simulink model "InjCtl_qCo1"  (R2016b)
settings: configuration reference "CodeGenConfigSet" (kept outside this file)
values from neighbouring files (symbols this model uses):
  FMA_qCor_C = Calibration.Parameter    [init_InjCtl_qCo.m]    (also in init_InjCtl_qCo_SIL.m = Simulink.Parameter)
  FMO_qCor_C = Calibration.Parameter    [init_InjCtl_qCo.m]    (also in init_InjCtl_qCo_SIL.m = Simulink.Parameter)
  InjCtl_swtDiffQntIn_C = Calibration.Parameter    [init_InjCtl_qCo.m]    (also in init_InjCtl_qCo_SIL.m = Simulink.Parameter)
undefined symbols (not defined in the file or in its folder): EngState_conv, Switch_conv
libraries: simulink x1
settings Model: Creator=lenovo  LastModifiedBy=zhoutinglin
settings ConfigSetRef: SourceLocation=Base Workspace

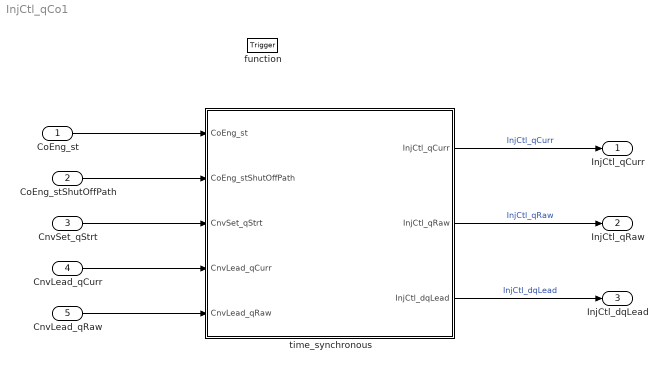
== system InjCtl_qCo1 ==
  CoEng_st : Inport  Description=Engine coordinator state  OutDataTypeStr=Enum: EngState_conv
  CoEng_stShutOffPath : Inport  Description=Active shut-off paths resulting from active reversible,irreversible and afterrun shut-off paths  Port=2  OutMin=0  OutMax=65535  OutDataTypeStr=State_uint16
  CnvSet_qStrt : Inport  Tag=mg/hub  Description=Injection start quantity  Port=3  OutMin=-319  OutMax=319  OutDataTypeStr=FuelMass_mg_hub
  CnvLead_qCurr : Inport  Tag=mg/hub  Description=Injection quantity current path  Port=4  OutMin=-319  OutMax=319  OutDataTypeStr=FuelMass_mg_hub
  CnvLead_qRaw : Inport  Tag=mg/hub  Description=Injection quantity raw path  Port=5  OutMin=-319  OutMax=319  OutDataTypeStr=FuelMass_mg_hub
  function : TriggerPort  TriggerType=function-call  VariantControl=Variant
  time_synchronous : Subsystem
  InjCtl_qCurr : Outport  Tag=mg/hub  Description=Torque generating engine fuel injection quantity  OutMin=-319  OutMax=319  OutDataTypeStr=FuelMass_mg_hub
  InjCtl_qRaw : Outport  Tag=mg/hub  Description=Raw value of injection mass  Port=2  OutMin=-319  OutMax=319  OutDataTypeStr=FuelMass_mg_hub
  InjCtl_dqLead : Outport  Tag=mg/hub  Description=Gradient of quantity  Port=3  OutMin=-319  OutMax=319  OutDataTypeStr=FuelMass_mg_hub
  wires:
  time_synchronous/1(InjCtl_qCurr) -> InjCtl_qCurr/1  "InjCtl_qCurr"
  time_synchronous/2(InjCtl_qRaw) -> InjCtl_qRaw/1  "InjCtl_qRaw"
  time_synchronous/3(InjCtl_dqLead) -> InjCtl_dqLead/1  "InjCtl_dqLead"
  CoEng_st/1 -> time_synchronous/1(CoEng_st)
  CoEng_stShutOffPath/1 -> time_synchronous/2(CoEng_stShutOffPath)
  CnvSet_qStrt/1 -> time_synchronous/3(CnvSet_qStrt)
  CnvLead_qCurr/1 -> time_synchronous/4(CnvLead_qCurr)
  CnvLead_qRaw/1 -> time_synchronous/5(CnvLead_qRaw)

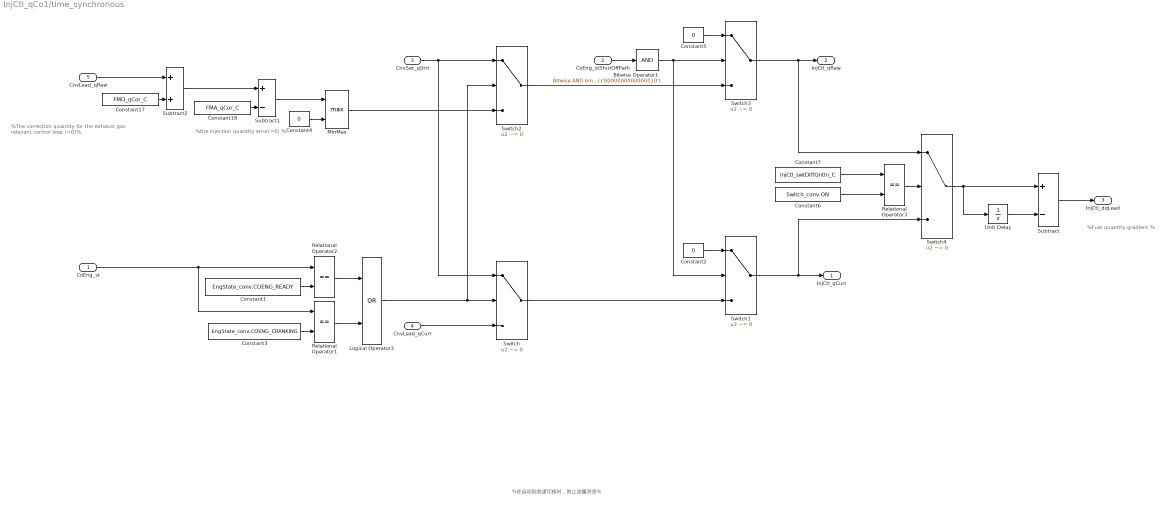
== system InjCtl_qCo1/time_synchronous ==
  note: %在启动到怠速切换时，防止油量突变%
  note: %Fuel quantity gradient %
  note: %The correction quantity for
      | the exhaust gas relevant control loop (=0)%
  note: %the injection quantity error(=0) %
  CoEng_st : Inport
  CoEng_stShutOffPath : Inport  Port=2
  CnvSet_qStrt : Inport  Port=3
  CnvLead_qCurr : Inport  Port=4
  CnvLead_qRaw : Inport  Port=5
  Bitwise Operator1 : simulink/Logic and Bit Operations/Bitwise Operator  logicop=AND  UseBitMask=on  BitMask=bin2dec('0000000000000010')  BitMaskRealWorld=Stored Integer
  Constant1 : Constant  Value=EngState_conv.COENG_READY
  Constant17 : Constant  Value=FMO_qCor_C  VectorParams1D=off
  Constant18 : Constant  Value=FMA_qCor_C  VectorParams1D=off
  Constant2 : Constant  Value=0  OutDataTypeStr=Inherit: Inherit via back propagation
  Constant3 : Constant  Value=EngState_conv.COENG_CRANKING
  Constant4 : Constant  Value=0  OutDataTypeStr=Inherit: Inherit via back propagation
  Constant5 : Constant  Value=0  OutDataTypeStr=Inherit: Inherit via back propagation
  Constant6 : Constant  Value=Switch_conv.ON
  Constant7 : Constant  Value=InjCtl_swtDiffQntIn_C  VectorParams1D=off
  Logical Operator3 : Logic  Operator=OR  AllPortsSameDT=off  OutDataTypeStr=boolean
  MinMax : MinMax  Function=max  Inputs=2
  Relational Operator1 : RelationalOperator  Operator===  OutDataTypeStr=boolean  RndMeth=Simplest  InputSameDT=on
  Relational Operator2 : RelationalOperator  Operator===  OutDataTypeStr=boolean  RndMeth=Simplest  InputSameDT=on
  Relational Operator3 : RelationalOperator  Operator===  OutDataTypeStr=boolean  RndMeth=Simplest  InputSameDT=on
  Subtract : Sum  Inputs=+-
  Subtract1 : Sum  Inputs=+-  OutDataTypeStr=Inherit: Inherit via back propagation  SaturateOnIntegerOverflow=on  InputSameDT=on
  Subtract2 : Sum  OutDataTypeStr=Inherit: Inherit via back propagation  SaturateOnIntegerOverflow=on  InputSameDT=on
  Switch{,1..4} (5 alike) : Switch  Criteria=u2 ~= 0  OutDataTypeStr=Inherit: Inherit via back propagation  SaturateOnIntegerOverflow=on  InputSameDT=on
  Unit Delay : UnitDelay  SampleTime=-1
  InjCtl_qCurr : Outport
  InjCtl_qRaw : Outport  Port=2
  InjCtl_dqLead : Outport  Port=3
  wires:
  Switch2/1 -> Switch3/3
  Logical Operator3/1 -> Switch2/2, Switch/2
  Bitwise Operator1/1 -> Switch3/2, Switch1/2
  Relational Operator3/1 -> Switch4/2
  Constant7/1 -> Relational Operator3/1
  Constant6/1 -> Relational Operator3/2
  Switch3/1 -> InjCtl_qRaw/1, Switch4/1
  Constant5/1 -> Switch3/1
  MinMax/1 -> Switch2/3
  Constant4/1 -> MinMax/2
  Subtract1/1 -> MinMax/1
  Constant18/1 -> Subtract1/2
  Constant17/1 -> Subtract2/2
  Subtract2/1 -> Subtract1/1
  CnvLead_qRaw/1 -> Subtract2/1
  CnvSet_qStrt/1 -> Switch2/1, Switch/1
  CnvLead_qCurr/1 -> Switch/3
  Switch1/1 -> InjCtl_qCurr/1, Switch4/3
  CoEng_stShutOffPath/1 -> Bitwise Operator1/1
  Constant2/1 -> Switch1/1
  Relational Operator2/1 -> Logical Operator3/1
  Constant1/1 -> Relational Operator2/2
  Relational Operator1/1 -> Logical Operator3/2
  CoEng_st/1 -> Relational Operator2/1, Relational Operator1/1
  Constant3/1 -> Relational Operator1/2
  Switch/1 -> Switch1/3
  Switch4/1 -> Unit Delay/1, Subtract/1
  Unit Delay/1 -> Subtract/2
  Subtract/1 -> InjCtl_dqLead/1
